simulink model "NonLinearControlTheoryHW1B"  (R2013a)
settings: Solver=ode45  StartTime=0.0  StopTime=25  RelTol=1e-3
settings Model: Creator=Samet  LastModifiedBy=Samet

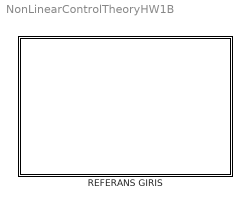
== system NonLinearControlTheoryHW1B ==
  REFERANS GIRIS : Subsystem
  wires:
  ? -> ?

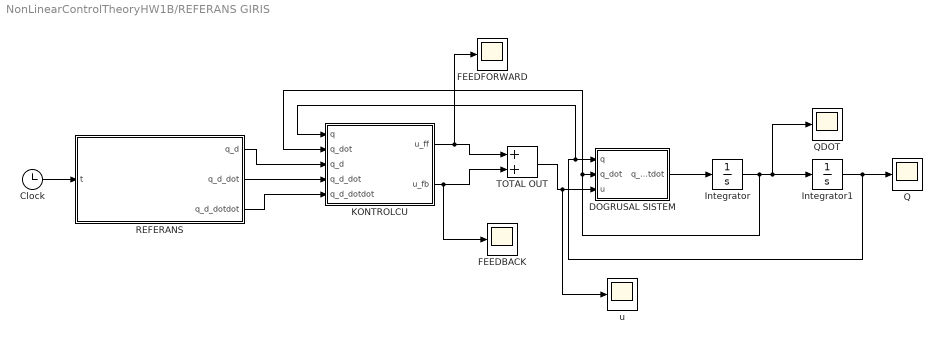
== system NonLinearControlTheoryHW1B/REFERANS GIRIS ==
  Clock : Clock
  DOGRUSAL SISTEM : MATLAB Function  TreatAsAtomicUnit=on
  FEEDBACK : Scope
      settings: TimeRange=10  YMin=-170  YMax=35
  FEEDFORWARD : Scope
  Integrator : Integrator
  Integrator1 : Integrator
  KONTROLCU : MATLAB Function  TreatAsAtomicUnit=on
  Q : Scope
      settings: TimeRange=10  SaveName=ScopeData3
  QDOT : Scope
      settings: TimeRange=10  YMax=8  SaveName=ScopeData4
  REFERANS : MATLAB Function  TreatAsAtomicUnit=on
  TOTAL OUT : Sum
  u : Scope
      settings: YMin=-170  YMax=40  SaveName=ScopeData2
  wires:
  Clock/1 -> REFERANS/1(t)
  REFERANS/3(q_d_dotdot) -> KONTROLCU/5(q_d_dotdot)
  REFERANS/2(q_d_dot) -> KONTROLCU/4(q_d_dot)
  REFERANS/1(q_d) -> KONTROLCU/3(q_d)
  KONTROLCU/1(u_ff) -> FEEDFORWARD/1, TOTAL OUT/1
  KONTROLCU/2(u_fb) -> TOTAL OUT/2, FEEDBACK/1
  DOGRUSAL SISTEM/1(q_dotdot) -> Integrator/1
  Integrator/1 -> QDOT/1, Integrator1/1, KONTROLCU/2(q_dot), DOGRUSAL SISTEM/2(q_dot)
  Integrator1/1 -> KONTROLCU/1(q), DOGRUSAL SISTEM/1(q), Q/1
  TOTAL OUT/1 -> u/1, DOGRUSAL SISTEM/3(u)

== matlab function NonLinearControlTheoryHW1B/REFERANS GIRIS/KONTROLCU ==
  data: q input; u_ff output; q_dot input; q_d input; q_d_dot input; q_d_dotdot input; u_fb output
function [u_ff,u_fb] = fcn(q,q_dot,q_d,q_d_dot,q_d_dotdot)
kv=1000;
kp=1000;
m=1.5;
e=q_d-q;
e_dot=q_d_dot-q_dot;
u_ff=m*q_d_dotdot;
u_fb=kv*e_dot+kp*e;

== matlab function NonLinearControlTheoryHW1B/REFERANS GIRIS/REFERANS ==
  data: t input; q_d output; q_d_dot output; q_d_dotdot output
function [q_d,q_d_dot,q_d_dotdot] = fcn(t)
q_d = 5+2*sin(t);
q_d_dot=2*cos(t);
q_d_dotdot=-2*sin(t);

== matlab function NonLinearControlTheoryHW1B/REFERANS GIRIS/DOGRUSAL SISTEM ==
  data: q input; q_dot input; u input; q_dotdot output
function q_dotdot = fcn(q,q_dot,u)
m=1.5;
b=2;
%q_dotdot =u/m;
q_dotdot=(u-(b*q*q_dot))/(m*(1+q^2));
